simulink library "adcs_main_lib"  (R2016b)
settings: Solver=VariableStepAuto  StartTime=0.0  StopTime=10.0  RelTol=1e-3
undefined symbols (not defined in the file): fsw_params
libraries: MSP_FSW_lib x1, MSP_env_estim x1
settings Model: Creator=taylorreynolds  LastModifiedBy=taylorreynolds

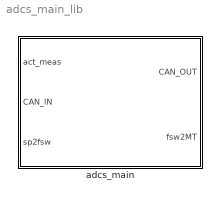
== system adcs_main_lib ==
  adcs_main : Subsystem

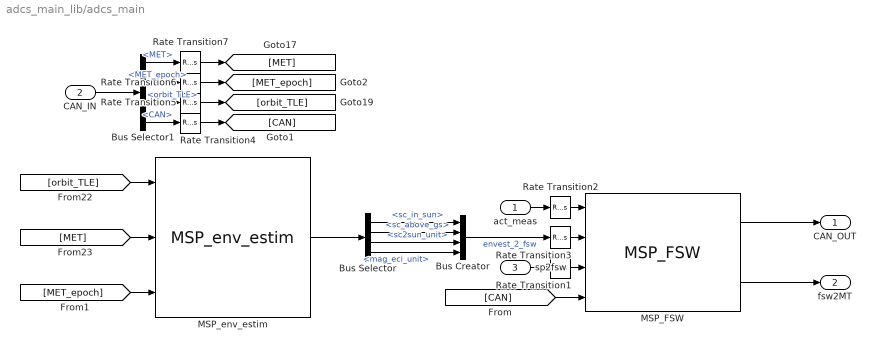
== system adcs_main_lib/adcs_main ==
  act_meas : Inport
  CAN_IN : Inport  Port=2  OutDataTypeStr=Bus: CAN_IN
  sp2fsw : Inport  Port=3  OutDataTypeStr=Bus: sp2fsw
  Bus Creator : BusCreator  Inputs=4
  Bus Selector : BusSelector  OutputSignals=sc_in_sun,sc_above_gs,sc2sun_unit,mag_eci_unit
  Bus Selector1 : BusSelector  OutputSignals=MET,MET_epoch,orbit_TLE,CAN
  MSP_FSW : MSP_FSW_lib/MSP_FSW
  MSP_env_estim : MSP_env_estim/MSP_env_estim
  Rate Transition{1..3,7} (4 alike) : RateTransition  OutPortSampleTime=fsw_params.sample_time_s
  Rate Transition4 : RateTransition  X0=fsw_params.bus.CAN_ic  OutPortSampleTime=fsw_params.sample_time_s
  Rate Transition5 : RateTransition  X0=fsw_params.bus.orbit_tle  OutPortSampleTime=fsw_params.sample_time_s
  Rate Transition6 : RateTransition  X0=fsw_params.bus.MET_epoch  OutPortSampleTime=fsw_params.sample_time_s
  CAN_OUT : Outport
  fsw2MT : Outport  Port=2
  wires:
  Rate Transition3/1 -> MSP_FSW/2
  Rate Transition7/1 -> [MET]
  Rate Transition6/1 -> [MET_epoch]
  Rate Transition5/1 -> [orbit_TLE]
  Rate Transition4/1 -> [CAN]
  CAN_IN/1 -> Bus Selector1/1
  Rate Transition1/1 -> MSP_FSW/3
  Rate Transition2/1 -> MSP_FSW/1
  [CAN] -> MSP_FSW/4
  Bus Selector1/4 -> Rate Transition4/1  "<CAN>"
  MSP_FSW/1 -> CAN_OUT/1
  sp2fsw/1 -> Rate Transition1/1
  MSP_env_estim/1 -> Bus Selector/1
  act_meas/1 -> Rate Transition2/1
  Bus Selector1/1 -> Rate Transition7/1  "<MET>"
  [MET] -> MSP_env_estim/2
  [orbit_TLE] -> MSP_env_estim/1
  Bus Selector1/3 -> Rate Transition5/1  "<orbit_TLE>"
  MSP_FSW/2 -> fsw2MT/1
  Bus Selector/1 -> Bus Creator/1  "<sc_in_sun>"
  Bus Selector/2 -> Bus Creator/2  "<sc_above_gs>"
  Bus Selector/3 -> Bus Creator/3  "<sc2sun_unit>"
  Bus Selector/4 -> Bus Creator/4  "<mag_eci_unit>"
  Bus Creator/1 -> Rate Transition3/1  "envest_2_fsw"
  Bus Selector1/2 -> Rate Transition6/1  "<MET_epoch>"
  [MET_epoch] -> MSP_env_estim/3
